simulink library "Susp_TwistBeam_Components"  (R2026a)
settings: Solver=VariableStepAuto
undefined symbols (not defined in the file): arm_mass, hp_arm, hp_beam, hp_shock_bot, hp_spr_bot, hp_whl_ctr, TwistBeam, Visual, X, Y, Z
libraries: Suspension_Utilities x4, sm_lib x2
Description:
  | Component of Simscape Vehicle Templates Library
  | 
  | Copyright 2018-2026 The MathWorks, Inc.
settings Model: Creator=mwalker  LastModifiedBy=smiller

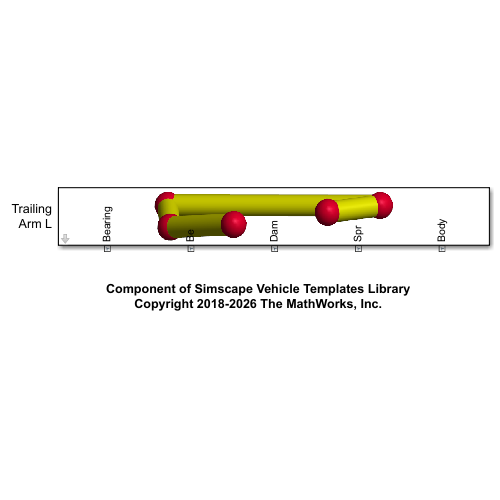
[thumbnail: Simulink's stored preview of the top-level diagram]
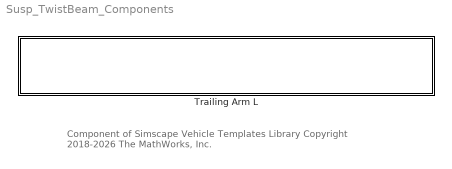
== system Susp_TwistBeam_Components ==
  note: Component of Simscape Vehicle Templates Library
      | Copyright 2018-2026 The MathWorks, Inc.
  Trailing Arm L : Subsystem  VariantControl=Steer  mask{popup_leftRight=Left, hp_body=hp_arm, hp_spr_bot=hp_spr_bot, hp_dam_bot=hp_shock_bot, hp_wctr=hp_whl_ctr, hp_beam=hp_beam, axle_whlc_to_bearing=TwistBeam.TrailingArm.xWCtoBearing.Value, rod_mass=arm_mass, clr_conn_rod=Visual.hp.clr, opc_conn_rod=Visual.hp.opc, size_conn_rod=Visual.hp.rad, clr_rod=Visual.UpperArm.clr, opc_rod=Visual.part.opc, radius_rod=Visual.UpperArm.rad}
      mask prompts: popup_leftRight "Left/Right"; hp_body "Body [xyz] (m)"; hp_spr_bot "Spring Bottom [xyz] (m)"; hp_dam_bot "Damper Bottom [xyz] (m)"; hp_wctr "Wheel Center [xyz] (m)"; hp_beam "Beam [xyz] (m)"; axle_whlc_to_bearing "Distance Wheel Ctr to Bearing (m)"; rod_mass "Mass (kg)"
      mask init:
      | if(popup_leftRight == 1)
      |     rhs_rod = 1;
      | elseif(popup_leftRight == 2)
      |     rhs_rod = -1;
      | end
      mask TypeOptions popup_leftRight: Left | Right
      mask TypeOptions rod_mass: Arm/Mass
      mask TypeOptions clr_conn_rod:
      | Vis
      | WCtr/GraphicDiffuseColor | Vis
      | Body/GraphicDiffuseColor
      mask TypeOptions opc_conn_rod:
      | Vis
      | WCtr/GraphicOpacity | Vis
      | Body/GraphicOpacity
      mask TypeOptions clr_rod: Arm/clr_solid
      mask TypeOptions opc_rod: Arm/opc_solid
      mask TypeOptions radius_rod: Arm/rad_solid
      mask DialogControl cont_arm Prompt: Arm
      mask DialogControl grp_rod Prompt: Part
      mask DialogControl cont_vis_rod Prompt: Visualization
      mask DialogControl text_clr_rod Prompt: Color [RGB]
      mask DialogControl text_opc_rod Prompt: Opac. (0-1)
      mask DialogControl text_size_rod Prompt: Size (m)
      mask DialogControl text_conn_rod Prompt: Connections
      mask DialogControl text_rod_rod Prompt: Rod
      mask Display: image('sm_car_vehicle_susp_twistbeam_trailingarm_IMAGE.png')

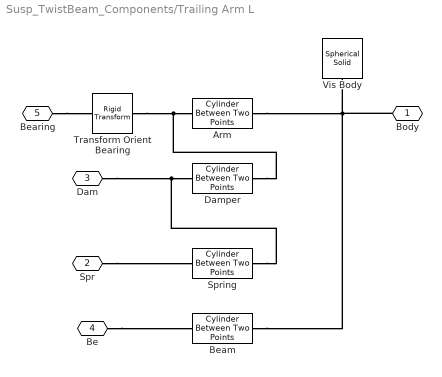
== system Susp_TwistBeam_Components/Trailing Arm L ==
  Arm : Suspension_Utilities/Cylinder Between Two Points  hp_b=hp_body.*[1 rhs_rod 1]  hp_f=hp_wctr.*[1 rhs_rod 1]-[0 axle_whlc_to_bearing 0].*[1 rhs_rod 1]  Mass=rod_mass  clr_solid=clr_rod  opc_solid=opc_rod  rad_solid=radius_rod
  Beam : Suspension_Utilities/Cylinder Between Two Points  hp_b=hp_body.*[1 rhs_rod 1]  hp_f=hp_beam.*[1 rhs_rod 1]  Mass=rod_mass  clr_solid=clr_rod  opc_solid=opc_rod  rad_solid=radius_rod
  Damper : Suspension_Utilities/Cylinder Between Two Points  hp_b=hp_wctr.*[1 rhs_rod 1]-[0 axle_whlc_to_bearing 0].*[1 rhs_rod 1]  hp_f=hp_dam_bot.*[1 rhs_rod 1]  Mass=rod_mass  clr_solid=clr_rod  opc_solid=opc_rod  rad_solid=radius_rod
  Spring : Suspension_Utilities/Cylinder Between Two Points  hp_b=hp_dam_bot.*[1 rhs_rod 1]  hp_f=hp_spr_bot.*[1 rhs_rod 1]  Mass=rod_mass  clr_solid=clr_rod  opc_solid=opc_rod  rad_solid=radius_rod
  Transform Orient Bearing : sm_lib/Frames and Transforms/Rigid Transform  RotationMethod=StandardAxis  FollAlignAxisA=+X  BaseAlignAxisA=+Y  FollAlignAxisB=+Y  BaseAlignAxisB=+Z  RotationStandardAxis=+X  RotationAngle=-90  RotationAngleUnits=deg  RotationArbitraryAxis=[0 0 1]  RotationSequenceAxes=FollowerAxes  RotationSequence=XYX  RotationSequenceAngles=[0 0 0]  RotationSequenceAnglesUnits=deg  RotationMatrix=[1 0 0; 0 1 0; 0 0 1]  Quaternion=[1 0 0 0]  TranslationMethod=None  TranslationCartesianOffset=[0 0 0]  TranslationCartesianOffsetUnits=m  TranslationStandardAxis=+Z  TranslationStandardOffset=0  TranslationStandardOffsetUnits=m  TranslationROffset=0  TranslationROffsetUnits=m  TranslationThetaOffset=0  TranslationThetaOffsetUnits=deg  TranslationZOffset=0  TranslationZOffsetUnits=m
  Vis Body : sm_lib/Body Elements/Spherical Solid  SphereRadius=size_conn_rod  SphereRadiusUnits=m  ExportEntireGeometry=off  InertiaType=CalculateFromGeometry  BasedOnType=Density  Density=0  DensityUnits=kg/m^3  Mass=1  MassUnits=kg  CenterOfMass=[0 0 0]  CenterOfMassUnits=m  MomentsOfInertia=[1 1 1]  MomentsOfInertiaUnits=kg*m^2  ProductsOfInertia=[0 0 0]  ProductsOfInertiaUnits=kg*m^2  GraphicType=FromGeometry  MarkerShape=Sphere  MarkerSize=10  GraphicVisPropType=SimpleVisualProperties  GraphicDiffuseColor=clr_conn_rod  GraphicOpacity=opc_conn_rod  GraphicSpecularColor=[0.5 0.5 0.5 1.0]  GraphicAmbientColor=[0.15 0.15 0.15 1.0]  GraphicEmissiveColor=[0.0 0.0 0.0 1.0]  GraphicShininess=75  DoExposeReferenceFrame=on  SerializedFrames=<Frames/>
  Body : PMIOPort  Side=Left
  Spr : PMIOPort  Port=2  Side=Left
  Dam : PMIOPort  Port=3  Side=Left
  Be : PMIOPort  Port=4  Side=Left
  Bearing : PMIOPort  Port=5  Side=Left
  connections:
  Body/RConn1 -- Arm/LConn1 -- Vis Body/RConn1 -- Beam/LConn1
  Spr/RConn1 -- Spring/RConn1
  Be/RConn1 -- Beam/RConn1
  Dam/RConn1 -- Spring/LConn1 -- Damper/RConn1
  Damper/LConn1 -- Transform Orient Bearing/LConn1 -- Arm/RConn1
  Bearing/RConn1 -- Transform Orient Bearing/RConn1
